simulink model "CAN_decoding"  (R2024b)
settings: Solver=FixedStepDiscrete  StartTime=startTime  StopTime=endTime  FixedStep=Ts  RelTol=1e-3  EnableMultiTasking=on
undefined symbols (not defined in the file or in its folder): canChannel
libraries: canlib x3, canmsglib x3
settings Model: Creator=elony  LastModifiedBy=elony

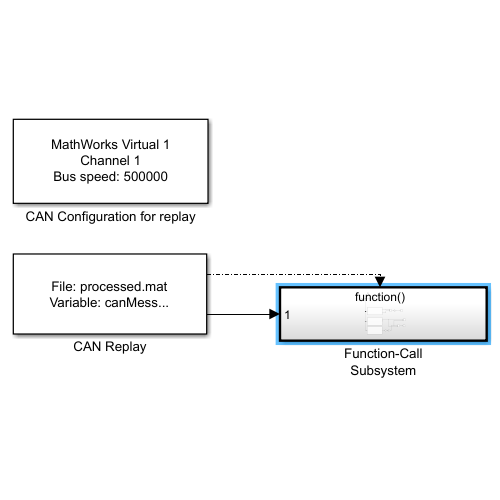
[thumbnail: Simulink's stored preview of the top-level diagram]
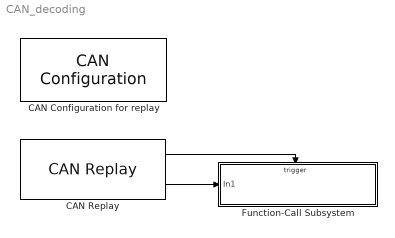
== system CAN_decoding ==
  CAN Configuration for replay : canlib/CAN Configuration  BlockHandle=154.0001  Device=MathWorks Virtual 1 (Channel 1)  DeviceMenu=MathWorks Virtual 1 (Channel 1)  ObjConstructor=canChannel('MathWorks', 'Virtual 1', 1)  BusSpeed=500000  EnableBitParameters=off  AckMode=Normal
  CAN Replay : canlib/CAN Replay  BlockHandle=155.0001  FullPathFileName=C:\Users\elony\OneDrive\Desktop\CAN_Hacking\CAN-message-Hacking\processed.mat  FileName=processed.mat  VariableName=canMessages  NoTimesReplay=Inf  ReplayTo=Output port  DeviceMenu=Select a device  Device=Select a device  ObjConstructor=Select a constructor  SampleTime=0.001  BusOutput=off
  Function-Call Subsystem : Subsystem  TreatAsAtomicUnit=on
  wires:
  CAN Replay/2 -> Function-Call Subsystem/1(In1)
  CAN Replay/1 -> Function-Call Subsystem/Trigger

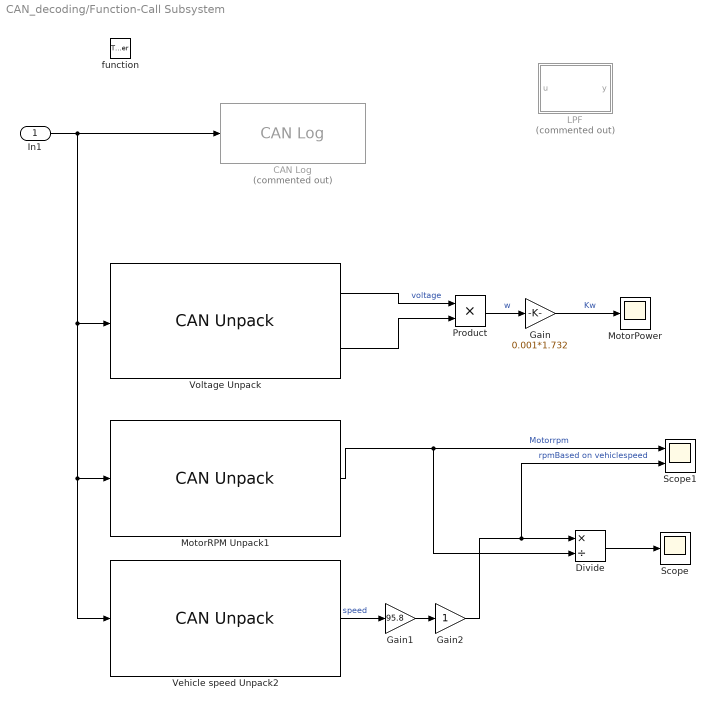
== system CAN_decoding/Function-Call Subsystem ==
  In1 : Inport
  function : TriggerPort  TriggerType=function-call  VariantControl=(inherit)
  CAN Log : canlib/CAN Log  Commented=on  BlockHandle=164.0001  FullPathFileName=C:\Users\elony\OneDrive\Desktop\CAN_Hacking\test.blf  FileName=test.blf  VariableName=current  MaxNumMessages=1000000  LogFrom=Input port  DeviceMenu=Select a device  Device=Select a device  ObjConstructor=Select a constructor  SampleTime=0.01
  Divide : Product  Inputs=*/
  Gain : Gain  Gain=0.001*1.732
  Gain1 : Gain  Gain=95.8
  Gain2 : Gain
  LPF : MATLAB Function  Commented=on  TreatAsAtomicUnit=on
  MotorPower : Scope
  MotorRPM Unpack1 : canmsglib/CAN Unpack  MsgList=(none)  MsgName=Vector__XXXMsg99  MsgIDType=Standard (11-bit identifier)  MsgIdentifier=0x108  MsgLength=8  SignalInfo={ 'RArpm', '40', '16', 'LE', 'signed', 'Standard', '0', '1.2', '0', '-2750', '2750' }  IDPort=off  TimestampPort=off  ErrorPort=off  RemotePort=off  LengthPort=off  StatusPort=off  ApplyMinMax=off
      settings: LibrarySourceBlock=canlib/CAN Unpack
  Product : Product
  Scope : Scope
  Scope1 : Scope  NumInputPorts=2
  Vehicle speed Unpack2 : canmsglib/CAN Unpack  MsgList=(none)  MsgName=Vehicle speed  MsgIDType=Standard (11-bit identifier)  MsgIdentifier=0x257  MsgLength=8  SignalInfo={ 'Vspeed', '24', '8', 'LE', 'unsigned', 'Standard', '0', '1', '0', '0', '255' }  IDPort=off  TimestampPort=off  ErrorPort=off  RemotePort=off  LengthPort=off  StatusPort=off  ApplyMinMax=off
      settings: LibrarySourceBlock=canlib/CAN Unpack
  Voltage Unpack : canmsglib/CAN Unpack  MsgList=(none)  MsgName=Vector__XXXMsg99  MsgIDType=Standard (11-bit identifier)  MsgIdentifier=0x126  MsgLength=8  SignalInfo={ 'Voltage', '0', '10', 'LE', 'unsigned', 'Standard', '0', '0.5', '0', '0', '1'; 'Current', '16', '10', 'LE', 'unsigned', 'Standard', '0', '1', '-1', '0', '1022' }  IDPort=off  TimestampPort=off  ErrorPort=off  RemotePort=off  LengthPort=off  StatusPort=off  ApplyMinMax=off
      settings: LibrarySourceBlock=canlib/CAN Unpack
  wires:
  In1/1 -> CAN Log/1, Vehicle speed Unpack2/1, MotorRPM Unpack1/1, Voltage Unpack/1
  Product/1 -> Gain/1  "w"
  Gain/1 -> MotorPower/1  "Kw"
  Voltage Unpack/1 -> Product/1  "voltage"
  Voltage Unpack/2 -> Product/2
  MotorRPM Unpack1/1 -> Divide/2, Scope1/1  "Motorrpm"
  Vehicle speed Unpack2/1 -> Gain1/1  "speed"
  Gain1/1 -> Gain2/1
  Gain2/1 -> Scope1/2, Divide/1  "rpmBased on vehiclespeed"
  Divide/1 -> Scope/1

== matlab function CAN_decoding/Function-Call Subsystem/LPF ==
  data: u input; y output
function y = fcn(u)
persistent lastOut
if isempty(lastOut),lastOut=0;end

y = u*0.02+lastOut*0.98;
lastOut=y;
end

%This low pass filter is changed from transfer fucntion of first order low
%pass filter. 
% rc=1/(2*pi*f_cutoff) filter coeffecient will be alpha=rc/(rc+Ts)
